simulink model "pos_test"  (Simulink 7.9)
settings: Solver=FixedStepDiscrete  StartTime=0.0  StopTime=60  FixedStep=ts  RelTol=1e-3
values from neighbouring files (symbols this model uses):
  ts = 1/50    (= 0.02)    [sim_init.m]    (also in sim_param.mat)
libraries: arduino_io_lib x5
settings Model: Creator=hirata  LastModifiedBy=hirata
settings DebuggingCC: FcnCallInpInsideContextMsg=Use local settings
settings GRTTargetCC: CombineOutputUpdateFcns=off  GRTInterface=on

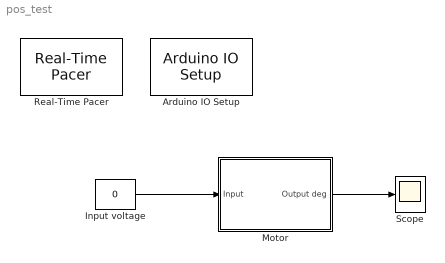
== system pos_test ==
  Arduino IO Setup : arduino_io_lib/Arduino IO Setup  Priority=3  arduinoVar=Temporary arduino variable: Arduino1  workspaceVarName=a  comPort=COM3
  Input voltage : Constant  Value=0
  Motor : Subsystem
  Real-Time Pacer : arduino_io_lib/Real-Time Pacer  simTimePerRealTime=1
  Scope : Scope
      settings: TimeRange=4  YMin=-120  YMax=120  SaveName=yout
  wires:
  Input voltage/1 -> Motor/1(Input)
  Motor/1(Output deg) -> Scope/1

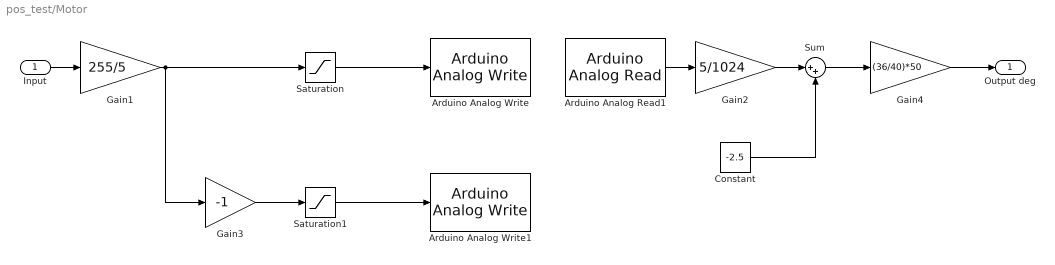
== system pos_test/Motor ==
  Input : Inport
  Arduino Analog Read1 : arduino_io_lib/Arduino Analog Read  arduinoVar=Temporary arduino variable: Arduino1  arduinoPin=0  T=ts
  Arduino Analog Write : arduino_io_lib/Arduino Analog Write  arduinoVar=Temporary arduino variable: Arduino1  arduinoPin=3  T=ts
  Arduino Analog Write1 : arduino_io_lib/Arduino Analog Write  arduinoVar=Temporary arduino variable: Arduino1  arduinoPin=5  T=ts
  Constant : Constant  Value=-2.5
  Gain1 : Gain  Gain=255/5
  Gain2 : Gain  Gain=5/1024
  Gain3 : Gain  Gain=-1
  Gain4 : Gain  Gain=(36/40)*50
  Saturation : Saturate  UpperLimit=255  LowerLimit=0
  Saturation1 : Saturate  UpperLimit=255  LowerLimit=0
  Sum : Sum  Inputs=|++
  Output deg : Outport
  wires:
  Input/1 -> Gain1/1
  Arduino Analog Read1/1 -> Gain2/1
  Saturation/1 -> Arduino Analog Write/1
  Gain1/1 -> Gain3/1, Saturation/1
  Saturation1/1 -> Arduino Analog Write1/1
  Gain4/1 -> Output deg/1
  Gain2/1 -> Sum/1
  Sum/1 -> Gain4/1
  Constant/1 -> Sum/2
  Gain3/1 -> Saturation1/1
